simulink model "Verifica_LQG_DE6000008"  (R2025b)
settings: Solver=VariableStepAuto  StartTime=0.0  StopTime=100.0  RelTol=1e-3
undefined symbols (not defined in the file): A, B, C, G, K_LQR_i, K_LQR_x, Qv, Rv, x0_sylv
libraries: cstblocks x1
settings Model: Creator=salvo  LastModifiedBy=salvo

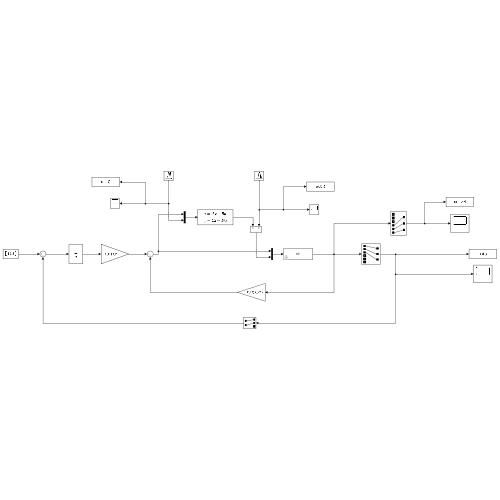
[thumbnail: Simulink's stored preview of the top-level diagram]
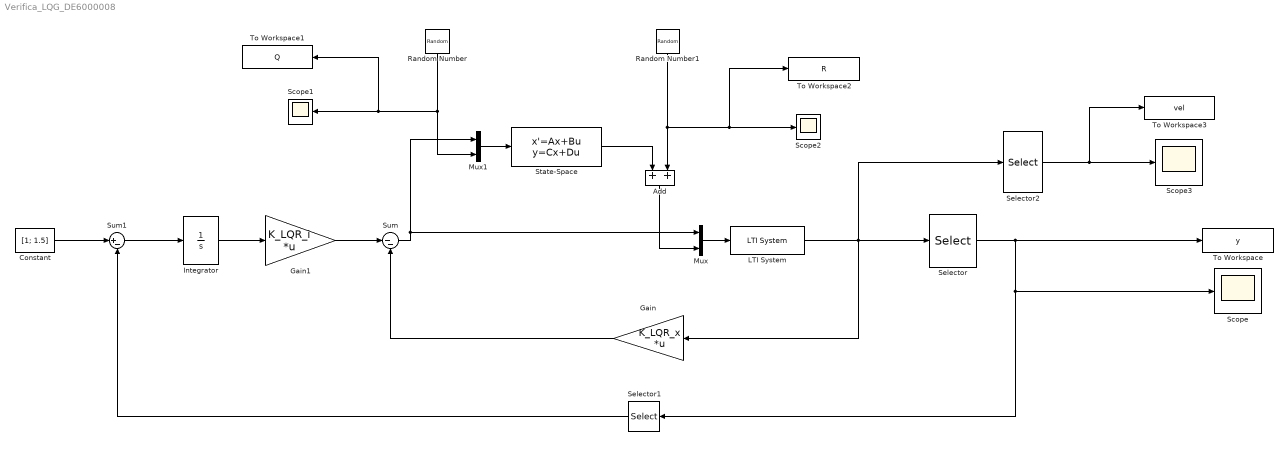
== system Verifica_LQG_DE6000008 ==
  Add : Sum
  Constant : Constant  Value=[1; 1.5]
  Gain : Gain  Gain=K_LQR_x  Multiplication=Matrix(K*u)
  Gain1 : Gain  Gain=K_LQR_i  Multiplication=Matrix(K*u)
  Integrator : Integrator
  LTI System : cstblocks/LTI System  sys=KF  IC=[]  PadeOrder=0
  Mux : Mux  Inputs=2
  Mux1 : Mux  Inputs=2
  Random Number : RandomNumber  Variance=diag(Qv)  SampleTime=0.1
  Random Number1 : RandomNumber  Variance=diag(Rv)  SampleTime=0.1
  Scope{,1..3} (4 alike) : Scope
      Scope settings: ActiveDisplayYMinimum=-2.5777000016596885  ActiveDisplayYMaximum=2.1067249142467013
      Scope1 settings: ActiveDisplayYMinimum=-1  ActiveDisplayYMaximum=1
      Scope2 settings: DataLoggingVariableName=ScopeData2
      Scope3 settings: ActiveDisplayYMinimum=-0.724818797682546  ActiveDisplayYMaximum=0.87655125593501171  DataLoggingVariableName=ScopeData3
  Selector : Selector  InputPortWidth=6  IndexOptions=Index vector (dialog)  Indices=[1 2 3]  OutputSizes=1
  Selector1 : Selector  InputPortWidth=3  IndexOptions=Index vector (dialog)  Indices=[1 2]  OutputSizes=1
  Selector2 : Selector  InputPortWidth=6  IndexOptions=Index vector (dialog)  Indices=[4 5 6]  OutputSizes=1
  State-Space : StateSpace  A=A  B=[B G]  C=C  D=zeros(3,8)  InitialCondition=x0_sylv
  Sum : Sum  Inputs=|--
  Sum1 : Sum  Inputs=|+-
  To Workspace : ToWorkspace  VariableName=y  SaveFormat=Timeseries  SampleTime=-1
  To Workspace1 : ToWorkspace  VariableName=Q  SaveFormat=Timeseries  SampleTime=-1
  To Workspace2 : ToWorkspace  VariableName=R  SaveFormat=Timeseries  SampleTime=-1
  To Workspace3 : ToWorkspace  VariableName=vel  SaveFormat=Timeseries  SampleTime=-1
  wires:
  Integrator/1 -> Gain1/1
  Gain/1 -> Sum/2
  Gain1/1 -> Sum/1
  Sum1/1 -> Integrator/1
  Selector/1 -> Selector1/1, Scope/1, To Workspace/1
  Constant/1 -> Sum1/1
  Mux1/1 -> State-Space/1
  Random Number1/1 -> To Workspace2/1, Scope2/1, Add/2
  State-Space/1 -> Add/1
  Random Number/1 -> To Workspace1/1, Scope1/1, Mux1/2
  Sum/1 -> Mux/1, Mux1/1
  Add/1 -> Mux/2
  Mux/1 -> LTI System/1
  LTI System/1 -> Selector2/1, Selector/1, Gain/1
  Selector1/1 -> Sum1/2
  Selector2/1 -> To Workspace3/1, Scope3/1
